simulink model "fault_injector"  (R2018b)
settings: Solver=VariableStepAuto  StartTime=0.0  StopTime=10.0  RelTol=1e-3
settings Model: Creator=jayakumarav  LastModifiedBy=hiterd
settings DebuggingCC: LibraryContextMissingDiagnostic=none
settings SFSimCC: SimUseLocalCustomCode=off
settings RTWCC: RTWUseLocalCustomCode=off

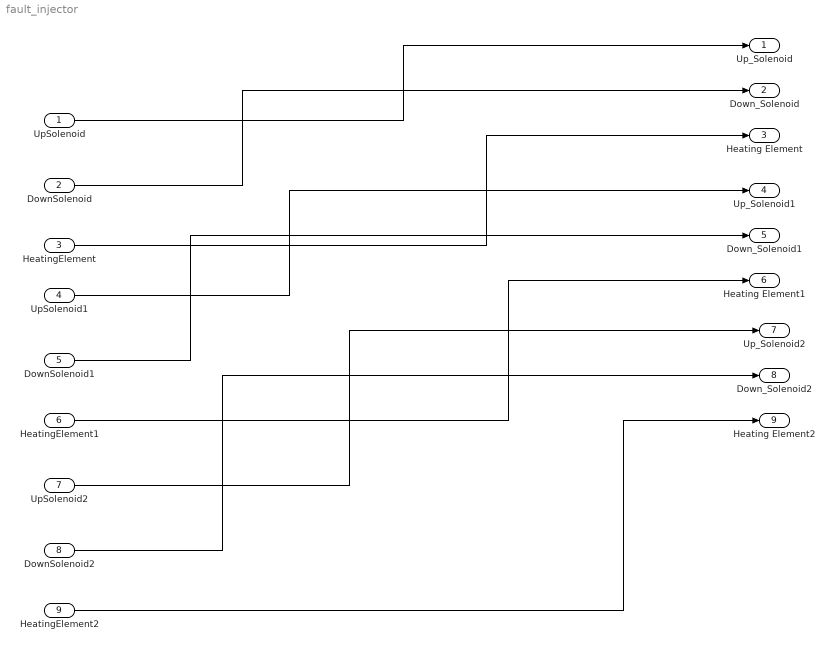
== system fault_injector ==
  UpSolenoid : Inport
  DownSolenoid : Inport  Port=2
  HeatingElement : Inport  Port=3
  UpSolenoid1 : Inport  Port=4
  DownSolenoid1 : Inport  Port=5
  HeatingElement1 : Inport  Port=6
  UpSolenoid2 : Inport  Port=7
  DownSolenoid2 : Inport  Port=8
  HeatingElement2 : Inport  Port=9
  Up_Solenoid : Outport
  Down_Solenoid : Outport  Port=2
  Heating Element : Outport  Port=3
  Up_Solenoid1 : Outport  Port=4
  Down_Solenoid1 : Outport  Port=5
  Heating Element1 : Outport  Port=6
  Up_Solenoid2 : Outport  Port=7
  Down_Solenoid2 : Outport  Port=8
  Heating Element2 : Outport  Port=9
  wires:
  UpSolenoid/1 -> Up_Solenoid/1
  DownSolenoid/1 -> Down_Solenoid/1
  HeatingElement/1 -> Heating Element/1
  UpSolenoid1/1 -> Up_Solenoid1/1
  DownSolenoid1/1 -> Down_Solenoid1/1
  HeatingElement1/1 -> Heating Element1/1
  UpSolenoid2/1 -> Up_Solenoid2/1
  DownSolenoid2/1 -> Down_Solenoid2/1
  HeatingElement2/1 -> Heating Element2/1
